simulink model "interactiveHarness"  (R2019b)
settings: Solver=FixedStepDiscrete  StartTime=0.0  StopTime=inf  FixedStep=Ts  MaxStep=Ts  RelTol=1e-3  EnableMultiTasking=on
libraries: simulink x1
settings Model: Creator=scastro  LastModifiedBy=bneiswan
settings SolverCC: MaxConsecutiveZCs=25
settings DataIOCC: DSMLogging=off  ReturnWorkspaceOutputs=off
settings OptimizationCC: DefaultParameterBehavior=Inlined  ExpressionDepthLimit=2147483647  InitFltsAndDblsToZero=on  LifeSpan=1  EfficientTunableParamExpr=on
settings DebuggingCC: UnderspecifiedInitializationDetection=Classic  MergeDetectMultiDrivingBlocksExec=none  ParameterPrecisionLossMsg=none  FcnCallInpInsideContextMsg=warning  AllowSymbolicDim=off  StateNameClashWarn=warning  PregeneratedLibrarySubsystemCodeDiagnostic=none  SFUnexpectedBacktrackingDiag=warning  SFNoUnconditionalDefaultTransitionDiag=warning  SFExecutionAtInitializationDiag=none  ArithmeticOperatorsInVariantConditions=warning
settings HardwareCC: ProdLongLongMode=on
settings ModelReferenceCC: UpdateModelReferenceTargets=IfOutOfDate  PropagateSignalLabelsOutOfModel=off
settings SFSimCC: SimUseLocalCustomCode=off  MATLABDynamicMemAlloc=off
settings RTWCC: SystemTargetFile=ert.tlc  TemplateMakefile=ert_default_tmf  RTWUseLocalCustomCode=off
settings CodeAppCC: IgnoreCustomStorageClasses=off  StateflowObjectComments=on
settings ERTTargetCC: MultiwordLength=2048  GenerateSampleERTMain=on  InlinedParameterPlacement=NonHierarchical  ERTCustomFileTemplate=example_file_process.tlc  ConvertIfToSwitch=off  SuppressUnreachableDefaultCases=off
settings ConfigComp: CovMetricSettings=dcmwe  CovHTMLOptions=-sRT=1 -sVT=0 -aTS=1 -bRG=1 -bTC=1 -hTR=0 -nFC=0 -nFD=1 -scm=1 -bcm=1 -xEv=0 -xEM=0  CovSaveCumulativeToWorkspaceVar=on  CovExternalEMLEnable=off  CovSFcnEnable=off  DVTestSuiteOptimization=CombinedObjectives (Nonlinear Extended)  DVIgnoreExistTestSatisfied=off  DVRebuildModelRepresentation=Always

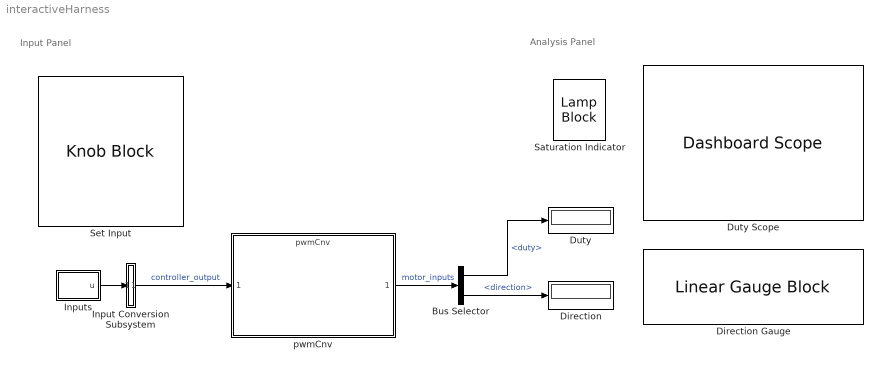
== system interactiveHarness ==
  note: Input Panel
  note: Analysis Panel
  Bus Selector : BusSelector  OutputSignals=duty,direction
  Direction : Display
  Direction Gauge : LinearGaugeBlock  ScaleMin=-2  ScaleMax=2  TickInterval=1
  Duty : Display
  Duty Scope : DashboardScope  TimeSpan=6000  Ymin=-1.1000000000000001  Ymax=1.1000000000000001  ScaleAtStop=off
  Input Conversion Subsystem : Subsystem  Tag=_input_conv_ss_
  Inputs : Subsystem
  Saturation Indicator : LampBlock  LabelPosition=Hide
  Set Input : KnobBlock  ScaleMin=-2  ScaleMax=2  TickInterval=0.5
  pwmCnv : ModelReference  ModelNameDialog=pwmCnv  SimulationMode=Normal  ModelReferenceVersion=1.185
  wires:
  Input Conversion Subsystem/1(Out_1) -> pwmCnv/1  "controller_output"
  pwmCnv/1 -> Bus Selector/1  "motor_inputs"
  Bus Selector/1 -> Duty/1  "<duty>"
  Bus Selector/2 -> Direction/1  "<direction>"
  Inputs/1(u) -> Input Conversion Subsystem/1(In_1)

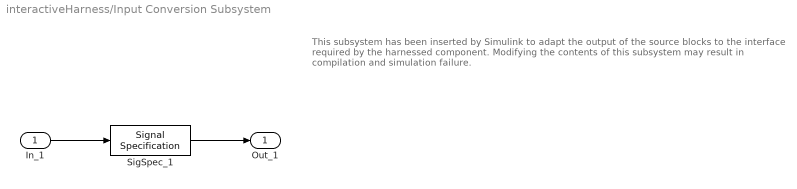
== system interactiveHarness/Input Conversion Subsystem ==
  note: This subsystem has been inserted by Simulink to adapt the output of the source blocks to the interface required by the harnessed component.
      |  Modifying the contents of this subsystem may result in compilation and simulation failure.
  In_1 : Inport
  SigSpec_1 : SignalSpecification  OutDataTypeStr=double  Dimensions=[1]  SampleTime=0.01
  Out_1 : Outport  VectorParamsAs1DForOutWhenUnconnected=off
  wires:
  In_1/1 -> SigSpec_1/1
  SigSpec_1/1 -> Out_1/1

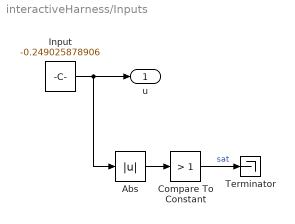
== system interactiveHarness/Inputs ==
  Abs : Abs
  Compare To Constant : simulink/Logic and Bit Operations/Compare To Constant  relop=>  const=1  OutDataTypeStr=boolean
  Input : Constant  Value=-0.249025878906
  Terminator : Terminator
  u : Outport  VectorParamsAs1DForOutWhenUnconnected=off
  wires:
  Input/1 -> u/1, Abs/1
  Compare To Constant/1 -> Terminator/1  "sat"
  Abs/1 -> Compare To Constant/1
